simulink model "InvertedPendulum_Simulink2018a"  (R2018a)
settings: Solver=ode4  StartTime=0.0  StopTime=SIM_TIME  FixedStep=STEP_SIZE  RelTol=1e-3
undefined symbols (not defined in the file): b, c, g, I, l, m, M, theta0, theta_dot0, x0, x_dot0
settings Model: Creator=roga  LastModifiedBy=roga
settings DataIOCC: ExternalInput=[0 0]  InitialState=[]  LoadExternalInput=on  LoadInitialState=on
settings OptimizationCC: DefaultParameterBehavior=Inlined  BufferReuse=off
settings DebuggingCC: AlgebraicLoopMsg=none  InitInArrayFormatMsg=none
settings SFSimCC: SimUseLocalCustomCode=on
settings RTWCC: RTWUseLocalCustomCode=on

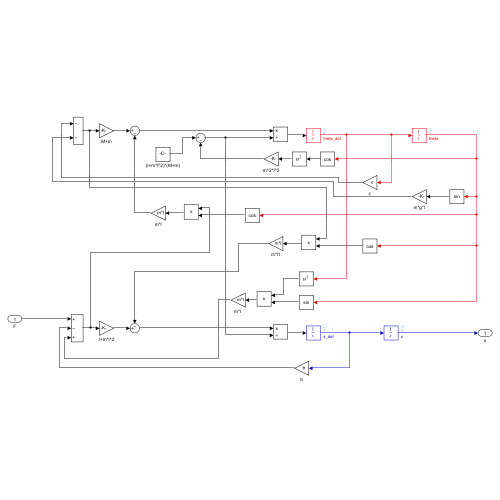
[thumbnail: Simulink's stored preview of the top-level diagram]
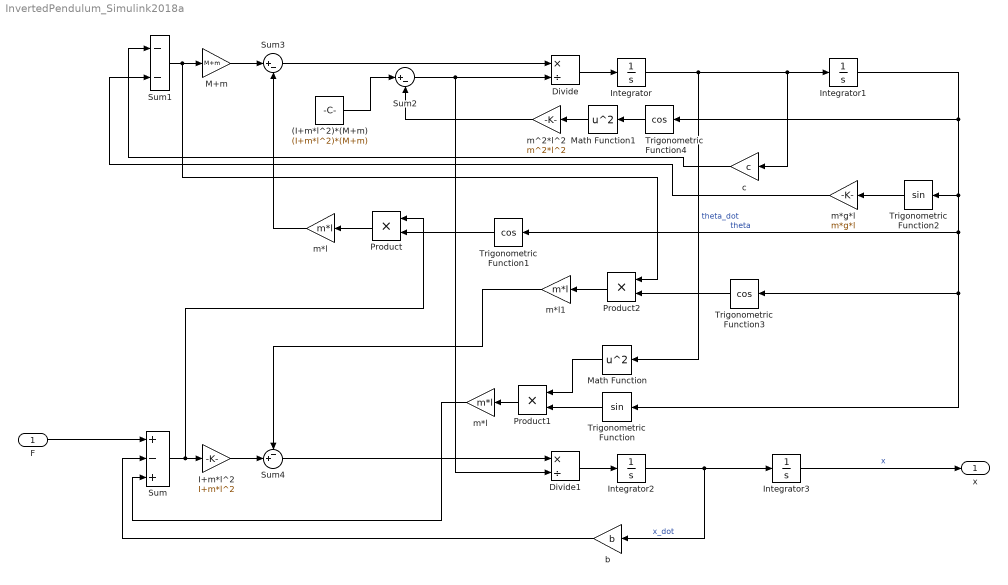
== system InvertedPendulum_Simulink2018a ==
  F : Inport
  (I+m*l^2)*(M+m) : Constant  Value=(I+m*l^2)*(M+m)
  Divide : Product  Inputs=*/
  Divide1 : Product  Inputs=*/
  I+m*l^2 : Gain  Gain=I+m*l^2
  Integrator : Integrator  Priority=1  InitialCondition=theta_dot0  ContinuousStateAttributes='pendulum.angular.velocity'
  Integrator1 : Integrator  Priority=2  InitialCondition=theta0  UpperSaturationLimit=pi  LowerSaturationLimit=-pi  ContinuousStateAttributes='pendulum.angular.position'
  Integrator2 : Integrator  Priority=3  InitialCondition=x_dot0  ContinuousStateAttributes='trolley.horizontal.velocity'
  Integrator3 : Integrator  Priority=4  InitialCondition=x0  ContinuousStateAttributes='trolley.horizontal.position'
  M+m : Gain  Gain=M+m
  Math Function : Math  Operator=square  SaturateOnIntegerOverflow=on
  Math Function1 : Math  Operator=square  SaturateOnIntegerOverflow=on
  Product : Product
  Product1 : Product
  Product2 : Product
  Sum : Sum  Inputs=+-+
  Sum1 : Sum  Inputs=--
  Sum2 : Sum  Inputs=|+-
  Sum3 : Sum  Inputs=|+-
  Sum4 : Sum  Inputs=-+|
  Trigonometric Function : Trigonometry
  Trigonometric Function1 : Trigonometry  Operator=cos
  Trigonometric Function2 : Trigonometry
  Trigonometric Function3 : Trigonometry  Operator=cos
  Trigonometric Function4 : Trigonometry  Operator=cos
  b : Gain  Gain=b
  c : Gain  Gain=c
  m*g*l : Gain  Gain=m*g*l
  m*l : Gain  Gain=m*l
  "m*l " : Gain  Gain=m*l
  m*l1 : Gain  Gain=m*l
  m^2*l^2 : Gain  Gain=m^2*l^2
  x : Outport
  wires:
  Integrator/1 -> Math Function/1, c/1, Integrator1/1  "theta_dot"
  Integrator2/1 -> b/1, Integrator3/1  "x_dot"
  Divide1/1 -> Integrator2/1
  F/1 -> Sum/1
  b/1 -> Sum/2
  Trigonometric Function1/1 -> Product/2
  Product/1 -> m*l/1
  Trigonometric Function/1 -> Product1/2
  Math Function/1 -> Product1/1
  Product1/1 -> "m*l "/1
  Trigonometric Function2/1 -> m*g*l/1
  Integrator1/1 -> Trigonometric Function4/1, Trigonometric Function2/1, Trigonometric Function1/1, Trigonometric Function3/1, Trigonometric Function/1  "theta"
  Integrator3/1 -> x/1  "x"
  c/1 -> Sum1/1
  m*g*l/1 -> Sum1/2
  Divide/1 -> Integrator/1
  Sum2/1 -> Divide1/2, Divide/2
  (I+m*l^2)*(M+m)/1 -> Sum2/1
  m^2*l^2/1 -> Sum2/2
  Trigonometric Function4/1 -> Math Function1/1
  Math Function1/1 -> m^2*l^2/1
  "m*l "/1 -> Sum/3
  Sum3/1 -> Divide/1
  M+m/1 -> Sum3/1
  m*l/1 -> Sum3/2
  Sum/1 -> Product/1, I+m*l^2/1
  I+m*l^2/1 -> Sum4/2
  Trigonometric Function3/1 -> Product2/2
  Product2/1 -> m*l1/1
  Sum1/1 -> Product2/1, M+m/1
  m*l1/1 -> Sum4/1
  Sum4/1 -> Divide1/1
